simulink library "VectorMagnitude_ul"  (R2020a)
settings: Solver=VariableStepAuto  StartTime=0.0  StopTime=10.0  RelTol=1e-3
settings Model: Creator=Ayaz  LastModifiedBy=Ayaz

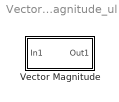
== system VectorMagnitude_ul ==
  Vector Magnitude : Subsystem

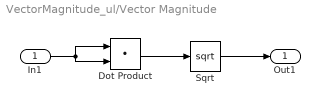
== system VectorMagnitude_ul/Vector Magnitude ==
  In1 : Inport
  Dot Product : DotProduct  InputSameDT=on  OutDataTypeStr=Inherit: Inherit via internal rule
  Sqrt : Sqrt  SaturateOnIntegerOverflow=on
  Out1 : Outport
  wires:
  In1/1 -> Dot Product/1, Dot Product/2
  Dot Product/1 -> Sqrt/1
  Sqrt/1 -> Out1/1
